simulink model "example3"  (Simulink 8.2)
settings: Solver=ode1  StartTime=0.0  StopTime=20  FixedStep=0.01  MaxStep=0.0001  RelTol=1e-5
undefined symbols (not defined in the file): DiscIntNeverNeededParam
settings Model: Creator=Jin  LastModifiedBy=Jin  PauseTimes=18
settings SolverCC: InitialStep=1e-5
settings DataIOCC: SignalLoggingSaveFormat=Dataset
settings OptimizationCC: ExpressionDepthLimit=128
settings DebuggingCC: FcnCallInpInsideContextMsg=EnableAllAsError  StateNameClashWarn=none
settings GRTTargetCC: CombineOutputUpdateFcns=on  GRTInterface=off

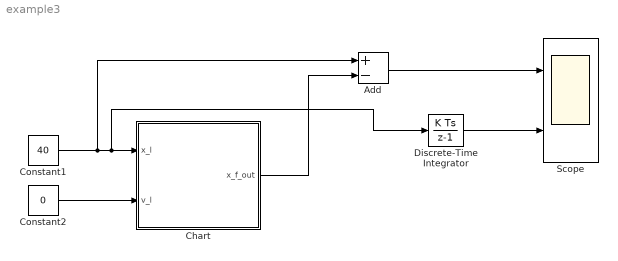
== system example3 ==
  Add : Sum  Inputs=+-
  Chart : Stateflow chart  TreatAsAtomicUnit=on
  Constant1 : Constant  Value=40
  Constant2 : Constant  Value=0
  Discrete-Time Integrator : DiscreteIntegrator  ICPrevOutput=DiscIntNeverNeededParam  ICPrevScaledInput=DiscIntNeverNeededParam
  Scope : Scope  NumInputPorts=2
      settings: YMin=-145~-5  YMax=-65~5
  wires:
  Add/1 -> Scope/1
  Constant1/1 -> Add/1, Discrete-Time Integrator/1, Chart/1(x_l)
  Constant2/1 -> Chart/2(v_l)
  Chart/1(x_f_out) -> Add/2
  Discrete-Time Integrator/1 -> Scope/2

== stateflow chart Chart ==
  settings: updateMethod=CONTINUOUS
  state Drive
    du:
    x_f_dot = 10;
    x_f_out = x_f;
  state Event
    du:
    x_f_dot = 0;
    x_f_out = x_f;
  (default) -> Drive : {x_f = 0;}
  Drive -> Event : [pow(x_l - x_f - 2, 0.5) <= 0]
  data: x_f local double; x_f_out output double; x_l input double; v_l input double
  data x_f settings: updateMethod=SF_CONTINUOUS_TIME_DATA
